simulink model "Jumping_Robot_system"  (R2019b)
settings: Solver=VariableStepAuto  StartTime=0.0  StopTime=10.0  RelTol=1e-3
PreLoadFcn:
  | set_parameters_JR.m
values from neighbouring files (symbols this model uses):
  g = 9.8    [set_parameters_JR.m]
  J_com_b = m_b*(H_body^2 + L_body^2)/12    (= 0.00510416666667)    [set_parameters_JR.m]
  J_m = 53.8e-7    (= 5.38e-06)    [set_parameters_JR.m]
  J_pivot_s = 0.33*m_s*H_spine^2    (= 0.0066825)    [set_parameters_JR.m]
  K = 10    [set_parameters_JR.m]
  l_s = H_spine/2    (= 0.225)    [set_parameters_JR.m]
  m_b = 2.5    [set_parameters_JR.m]
  m_s = 0.1    [set_parameters_JR.m]
  p_b = L_body/4    (= 0.035)    [set_parameters_JR.m]
  r = 1e-3    (= 0.001)    [set_parameters_JR.m]
Description:
  | Simulation of the Jumping Robot.  The dynamics are created with symbolic manipulation in Matlab.
settings Model: Creator=ecolgate  LastModifiedBy=ecolgate

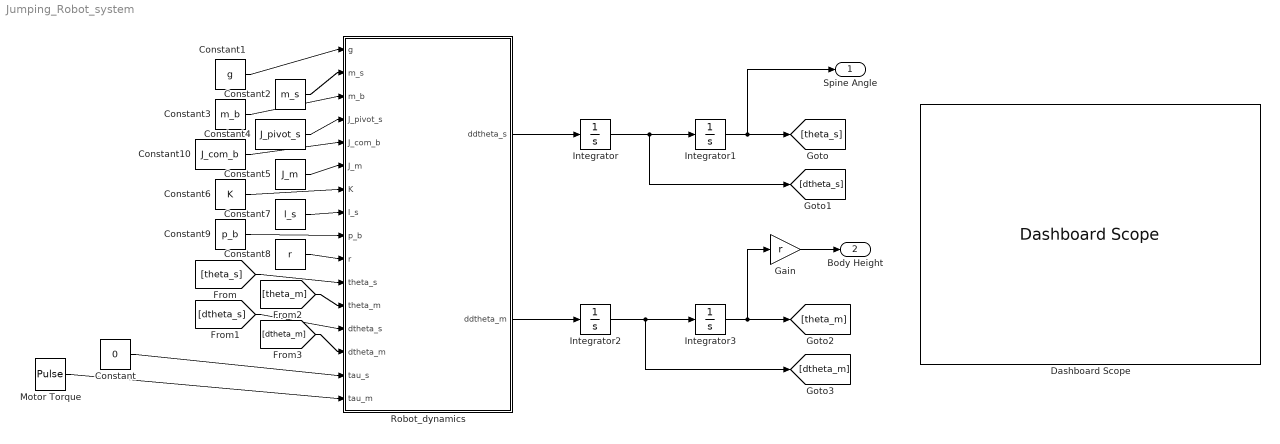
== system Jumping_Robot_system ==
  Constant : Constant  Value=0
  Constant1 : Constant  Value=g
  Constant10 : Constant  Value=J_com_b
  Constant2 : Constant  Value=m_s
  Constant3 : Constant  Value=m_b
  Constant4 : Constant  Value=J_pivot_s
  Constant5 : Constant  Value=J_m
  Constant6 : Constant  Value=K
  Constant7 : Constant  Value=l_s
  Constant8 : Constant  Value=r  VectorParams1D=off
  Constant9 : Constant  Value=p_b
  Dashboard Scope : DashboardScope  TimeSpan=1
  Gain : Gain  Gain=r
  Integrator{,1..3} (4 alike) : Integrator
  Motor Torque : DiscretePulseGenerator  PulseType=Time based  Amplitude=.15  Period=1  PulseWidth=30
  Robot_dynamics : MATLAB Function  TreatAsAtomicUnit=on
  Spine Angle : Outport
  Body Height : Outport  Port=2
  wires:
  Robot_dynamics/1(ddtheta_s) -> Integrator/1
  Robot_dynamics/2(ddtheta_m) -> Integrator2/1
  Integrator2/1 -> [dtheta_m], Integrator3/1
  Integrator/1 -> [dtheta_s], Integrator1/1
  [theta_s] -> Robot_dynamics/11(theta_s)
  Integrator1/1 -> Spine Angle/1, [theta_s]
  [dtheta_s] -> Robot_dynamics/13(dtheta_s)
  Integrator3/1 -> Gain/1, [theta_m]
  [theta_m] -> Robot_dynamics/12(theta_m)
  [dtheta_m] -> Robot_dynamics/14(dtheta_m)
  Constant/1 -> Robot_dynamics/15(tau_s)
  Motor Torque/1 -> Robot_dynamics/16(tau_m)
  Constant8/1 -> Robot_dynamics/10(r)
  Constant9/1 -> Robot_dynamics/9(p_b)
  Constant7/1 -> Robot_dynamics/8(l_s)
  Constant6/1 -> Robot_dynamics/7(K)
  Constant5/1 -> Robot_dynamics/6(J_m)
  Constant10/1 -> Robot_dynamics/5(J_com_b)
  Constant3/1 -> Robot_dynamics/3(m_b)
  Constant2/1 -> Robot_dynamics/2(m_s)
  Constant1/1 -> Robot_dynamics/1(g)
  Constant4/1 -> Robot_dynamics/4(J_pivot_s)
  Gain/1 -> Body Height/1

== matlab function Jumping_Robot_system/Robot_dynamics ==
  data: g input; ddtheta_s output; m_s input; m_b input; J_pivot_s input; J_com_b input; J_m input; K input; l_s input; p_b input; r input; theta_s input; theta_m input; dtheta_s input; dtheta_m input; tau_s input; tau_m input; ddtheta_m output
function [ddtheta_s,ddtheta_m] = Robot_dynamics(g,m_s,m_b,J_pivot_s,J_com_b,J_m,K,l_s,p_b,r,theta_s,theta_m,dtheta_s,dtheta_m,tau_s,tau_m)
%#codegen

%    This function was generated by the Symbolic Math Toolbox version 8.4.
%    03-Apr-2020 12:38:52

t2 = cos(theta_s);
t3 = sin(theta_s);
t4 = K.*theta_s;
t5 = dtheta_s.^2;
t6 = m_b.^2;
t7 = p_b.^2;
t8 = r.^2;
t10 = theta_m.^2;
t11 = J_com_b.*J_m;
t12 = J_m.*J_pivot_s;
t14 = m_b.*p_b.*r;
t15 = theta_s-1.0;
t9 = t8.^2;
t13 = g.*t2;
t16 = -t4;
t17 = sin(t15);
t18 = r.*t5.*theta_m;
t20 = -t14;
t21 = J_m.*m_b.*t7;
t22 = J_com_b.*m_b.*t8;
t23 = J_m.*m_b.*t8;
t24 = J_pivot_s.*m_b.*t8;
t25 = J_m.*t14.*2.0;
t26 = g.*m_b.*r.*t3.*theta_m;
t31 = dtheta_m.*dtheta_s.*m_b.*t8.*theta_m.*2.0;
t19 = m_b.*p_b.*t13;
t27 = -t18;
t28 = J_m+t20;
t30 = t10.*t23;
t32 = g.*l_s.*m_s.*t17;
t33 = t6.*t9.*t10;
t34 = -t31;
t29 = -t19;
t35 = t13+t27;
t40 = t11+t12+t21+t22+t23+t24+t25+t30+t33;
t36 = m_b.*r.*t35;
t39 = t16+t26+t29+t32+t34+tau_s;
t41 = 1.0./t40;
ddtheta_s = -t28.*t41.*(t36-tau_m)-t41.*(J_m+m_b.*t8).*(t4+t19-t26+t31-t32-tau_s);
if nargout > 1
    ddtheta_m = -t28.*t41.*(t4+t19-t26+t31-t32-tau_s)-t41.*(t36-tau_m).*(J_com_b+J_m+J_pivot_s+m_b.*t7+m_b.*t8.*t10);
end
